simulink model "BMS_Full_Model"  (R2024a)
settings: Solver=VariableStepAuto  StartTime=0.0  StopTime=3600  RelTol=1e-3
undefined symbols (not defined in the file): Ion, Lithium
libraries: spsParallelRLCBranchLib x9, spsMosfetLib x9, spsBatteryLib x8, spsIdealSwitchLib x4, spsControlledCurrentSourceLib x1, spsDCVoltageSourceLib x1, spsDiodeLib x1, spsDCMachineLib x1, sps_lib x1, spsVoltageMeasurementLib x1
settings Model: Creator=kanna  LastModifiedBy=kanna

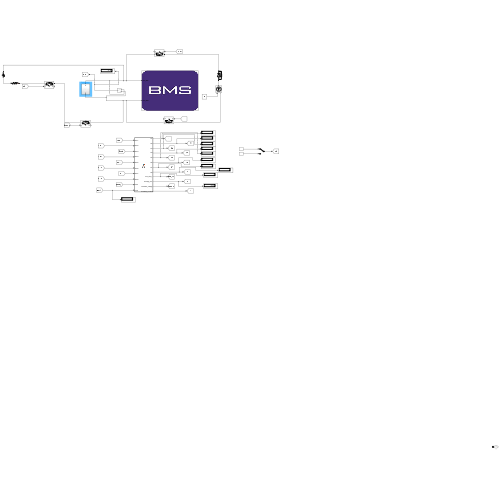
[thumbnail: Simulink's stored preview of the top-level diagram]
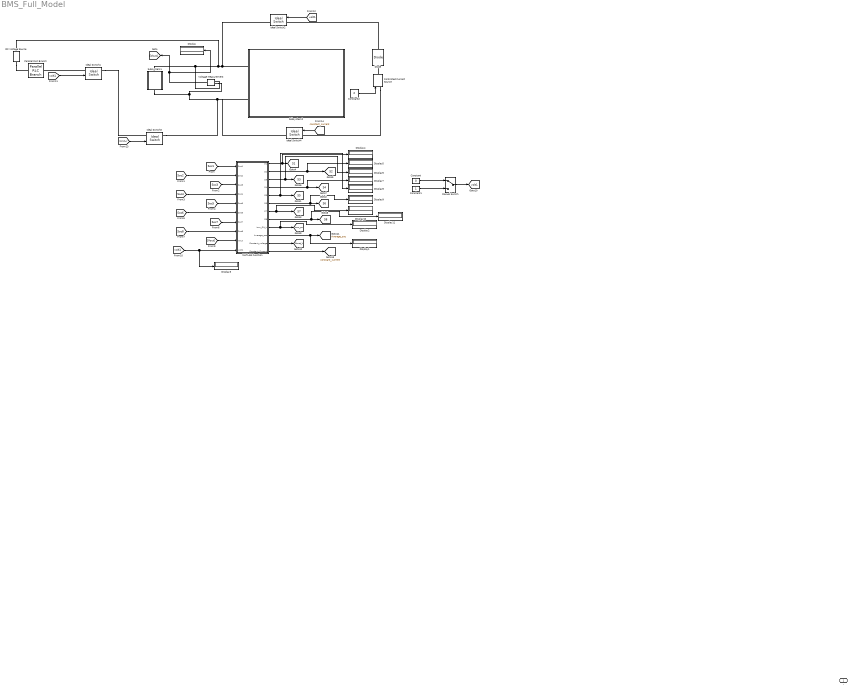
== system BMS_Full_Model ==
  Constant : Constant  Value=0
  Constant1 : Constant
  Constant2 : Constant  Value=2
  Controlled Current Source : spsControlledCurrentSourceLib/Controlled Current Source  Initialize=on  Source_Type=AC  Amplitude=0  Phase=0  Frequency=0  Measurements=None
  DC Voltage Source : spsDCVoltageSourceLib/DC Voltage Source  Amplitude=35  Measurements=None
  Diode : spsDiodeLib/Diode  Ron=0.001  Lon=0  Vf=0.8  IC=0  UseSnubber=0  Rs=500  Cs=250e-9  Measurements=off
  Display{,1..11} (12 alike) : Display
  Ideal Switch{1..4} (4 alike) : spsIdealSwitchLib/Ideal Switch  Ron=0.001  Lon=0  IC=0  Rs=1e5  Cs=inf  Measurements=on
  MATLAB Function : MATLAB Function  TreatAsAtomicUnit=on
  Manual Switch : ManualSwitch
  Parallel RLC Branch : spsParallelRLCBranchLib/Parallel RLC Branch  LConnTagsString=a  RConnTagsString=__new0  BranchType=R  Resistance=0.01  Inductance=1e-3  SetiL0=off  InitialCurrent=0  Capacitance=1e-6  Setx0=off  InitialVoltage=0  Measurements=None
  Subsystem1 : Subsystem
      settings: PortSchema="{\"entries\":[{\"content\":{\"sides\":[{\"content\":{},\"type\":\"ConnectorPlacement.EquallySpacedRectSide\",\"uuid\":\"ddaecf03-398d-4abe-ba2f-3d259c6a364a\"},{\"content\":{\"side\":\"RIGHT\"},\"type\":\"ConnectorPlacement.EquallySpacedRectSide\",\"uuid\":\"4de1636c-7844-41eb-a09b-b1e66b59fa18\"},{\"content\":{\"connectorIds\":[\"LConn1\"],\"side\":\"TOP\"},\"type\":\"ConnectorPlacement.EquallySpacedRectSide\",\"uuid\":\"76f54170-5ad1-4ec7-8870-ed8c99fdcc66\"},{\"content\":{\"connectorIds\":[\"RConn1\"],\"side\":\"BOTTOM\"},\"type\":\"ConnectorPlacement.EquallySpacedRectSide\",\"uuid\":\"75862763-7556-4715-9241-6073651da05c\"}]},\"type\":\"ConnectorPlacement.EquallySpacedConnector\",\"uuid\":\"7b1f8564-d695-4f68-8303-aa99595362ac\"}],\"packageUris\":[\"http://schema.mathworks.com/mf0/Connector/R2020b\"],\"version\":\"1.0\"}"
  Subsystem2 : Subsystem
      mask Display: image('GV4MPz3W8AAKAQj.jpeg');
  Voltage Measurement : spsVoltageMeasurementLib/Voltage Measurement  PhasorSimulation=off  OutputType=Complex  PSBequivalent=0
  - : PMIOPort  Side=Left
  tag scope: Average_soc=global, Const_V=global, S1=global, S2=global, S3=global, S4=global, S5=global, S6=global, S7=global, S8=global, constant_current=global, turn_on=global, volt1=global
  wires:
  MATLAB Function/1(S1) -> Display4/1, [S1]
  [Soc1] -> MATLAB Function/1(Soc1)
  [Soc2] -> MATLAB Function/2(Soc2)
  [Soc3] -> MATLAB Function/3(Soc3)
  [Soc4] -> MATLAB Function/4(Soc4)
  [Soc5] -> MATLAB Function/5(Soc5)
  [Soc6] -> MATLAB Function/6(Soc6)
  [Soc7] -> MATLAB Function/7(Soc7)
  [Soc8] -> MATLAB Function/8(Soc8)
  MATLAB Function/2(S2) -> Display5/1, [S2]
  MATLAB Function/3(S3) -> Display6/1, [S3]
  MATLAB Function/4(S4) -> Display7/1, [S4]
  MATLAB Function/5(S5) -> Display8/1, [S5]
  MATLAB Function/6(S6) -> Display9/1, [S6]
  MATLAB Function/7(S7) -> Display10/1, [S7]
  MATLAB Function/8(S8) -> Display11/1, [S8]
  Voltage Measurement/1 -> [Vout], Display/1
  [Vout] -> MATLAB Function/9(Vout)
  MATLAB Function/9(turn_ON_L) -> Display2/1, [turn_on]
  Constant/1 -> Manual Switch/1
  Constant1/1 -> Manual Switch/2
  [volt1] -> Ideal Switch1/1
  [volt1] -> Ideal Switch2/1
  MATLAB Function/10(Average_soc) -> Display1/1, [Average_soc]
  MATLAB Function/11(Constant_voltage) -> [Const_V]
  MATLAB Function/12(Constant_Current) -> [constant_current]
  [volt1] -> Display3/1, MATLAB Function/10(volt1)
  [Const_V] -> Ideal Switch3/1
  [constant_current] -> Ideal Switch4/1
  Manual Switch/1 -> [volt1]
  Constant2/1 -> Controlled Current Source/1
  connections:
  Ideal Switch1/LConn1 -- Parallel RLC Branch/LConn1
  DC Voltage Source/RConn1 -- Parallel RLC Branch/RConn1
  Ideal Switch2/RConn1 -- Subsystem2/LConn1 -- DC Voltage Source/LConn1 -- Subsystem1/RConn1 -- Voltage Measurement/LConn2
  Ideal Switch1/RConn1 -- Ideal Switch3/LConn1
  Controlled Current Source/LConn1 -- Ideal Switch4/LConn1
  Controlled Current Source/RConn1 -- Diode/LConn1
  Diode/RConn1 -- Ideal Switch2/LConn1
  Voltage Measurement/LConn1 -- Subsystem1/LConn1 -- Subsystem2/LConn2 -- Ideal Switch4/RConn1 -- Ideal Switch3/RConn1

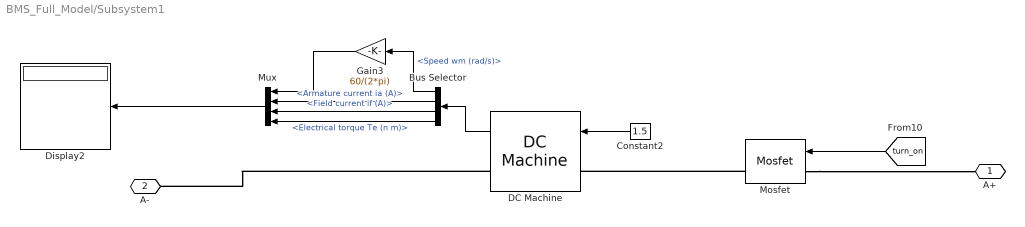
== system BMS_Full_Model/Subsystem1 ==
  Bus Selector : BusSelector  OutputSignals=Speed wm (rad/s),Armature current ia (A),Field current if (A),Electrical torque Te (n m)
  Constant2 : Constant  Value=1.5
  DC Machine : spsDCMachineLib/DC Machine  PresetModel=No  MechanicalLoad=Torque TL  FieldType=Permanent magnet  ShowDetailedParameters=on  MeasurementBus=off  RLa="[ 0.6  0.012]"  RLf="[ 240  120]"  Laf=1.8  MachineConstant=Torque constant (N.m/A)  Ke=1.8  Kt=1.8  J=1  Bm=0  Tf=0  w0=1  Ifinit=1.23834839145192e-21  TsPowergui=0  TsBlock=-1
  Display2 : Display
  Gain3 : Gain  Gain=60/(2*pi)
  Mosfet : spsMosfetLib/Mosfet  Ron=0.1  Lon=0  Rd=0.01  Vfd=0  IC=0  Rs=1e5  Cs=inf  Measurements=on
  Mux : Mux
  A+ : PMIOPort  Side=Left
  A- : PMIOPort  Port=2  Side=Right
  wires:
  Mux/1 -> Display2/1
  Gain3/1 -> Mux/1
  Bus Selector/4 -> Mux/4  "<Electrical torque Te (n m)>"
  Bus Selector/3 -> Mux/3  "<Field current if (A)>"
  Bus Selector/2 -> Mux/2  "<Armature current ia (A)>"
  Bus Selector/1 -> Gain3/1  "<Speed wm (rad/s)>"
  DC Machine/1 -> Bus Selector/1
  Constant2/1 -> DC Machine/1
  [turn_on] -> Mosfet/1
  connections:
  DC Machine/RConn1 -- A-/RConn1
  Mosfet/LConn1 -- A+/RConn1
  Mosfet/RConn1 -- DC Machine/LConn1

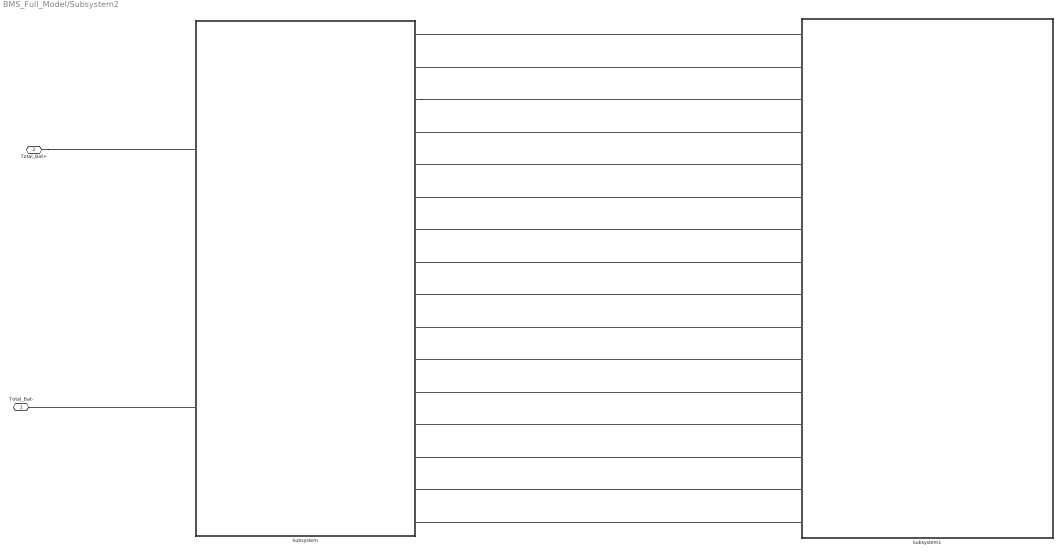
== system BMS_Full_Model/Subsystem2 ==
  Subsystem : Subsystem
  Subsystem1 : Subsystem
  Total_Bat- : PMIOPort  Side=Left
  Total_Bat+ : PMIOPort  Port=2  Side=Left
  connections:
  Total_Bat+/RConn1 -- Subsystem/LConn1
  Subsystem/LConn2 -- Total_Bat-/RConn1
  Subsystem1/LConn16 -- Subsystem/RConn16
  Subsystem1/LConn15 -- Subsystem/RConn15
  Subsystem1/LConn14 -- Subsystem/RConn14
  Subsystem1/LConn13 -- Subsystem/RConn13
  Subsystem1/LConn12 -- Subsystem/RConn12
  Subsystem1/LConn11 -- Subsystem/RConn11
  Subsystem1/LConn10 -- Subsystem/RConn10
  Subsystem1/LConn9 -- Subsystem/RConn9
  Subsystem1/LConn8 -- Subsystem/RConn8
  Subsystem1/LConn7 -- Subsystem/RConn7
  Subsystem1/LConn6 -- Subsystem/RConn6
  Subsystem1/LConn5 -- Subsystem/RConn5
  Subsystem1/LConn4 -- Subsystem/RConn4
  Subsystem1/LConn2 -- Subsystem/RConn2
  Subsystem1/LConn1 -- Subsystem/RConn1
  Subsystem/RConn3 -- Subsystem1/LConn3

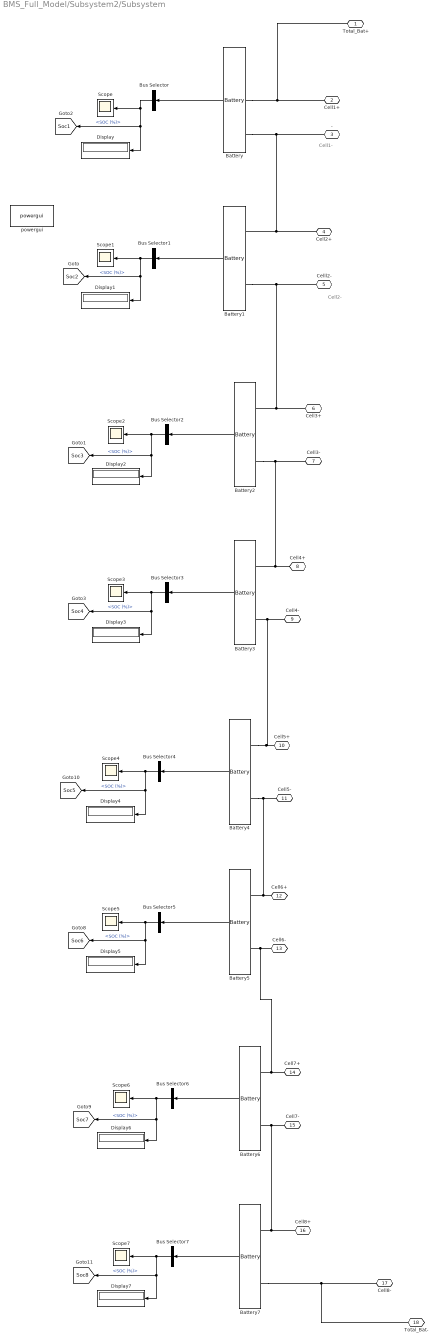
== system BMS_Full_Model/Subsystem2/Subsystem ==
  note: Cell2-
  note: Cell1-
  Battery : spsBatteryLib/Battery  BatType=Lithium-Ion  ShowTempParam=on  ThermalPreset="3.3V  2.3Ah  (LiFePO4)"  ShowAgeParam=off  NomV=3.3  NomQ=2.3  SOC=100  Batt_Tr=30  PresetModel=off  MaxQ=2.3  MinV=2.475  FullV=3.748  Dis_rate=2.3  R=0.014  Normal_OP=2.25  expZone="[3.4788       0.113]"  current=[6.5 13 32.5]  Units=Time  Tci=20  NomT=25  T2=0  MaxQ2=2.208  FullV2=3.45  Normal_OP2=2.85  expZone2="[3.22       0.015]"  Rca=0.6  ti=1000  Dp=0  Neq0=0  Tsim=1e6  Ta1=25  Qeol=5.4*0.9  Reol=0.013333*1.2  Char_age=[2.3478, 3]  Dis_age=[2.3478, 10]  N1=1500  N2=10500  N3=1000  N4=1400  Ta2=45  N5=950
  Battery{1..2,5..7} (5 alike) : spsBatteryLib/Battery  BatType=Lithium-Ion  ShowTempParam=off  ThermalPreset=no  ShowAgeParam=off  NomV=3.2  NomQ=18  SOC=100  Batt_Tr=30  PresetModel=on  MaxQ=18  MinV=2.4  FullV=3.7248  Dis_rate=7.8261  R=0.0017778  Normal_OP=16.2783  expZone="[3.4572     0.88435]"  current=[6.5 13 32.5]  Units=Time  Tci=20  NomT=20  T2=-30  MaxQ2=4.8  FullV2=7.1  Normal_OP2=5.655  expZone2="[6.58           1]"  Rca=0.6  ti=2000  Dp=0  Neq0=0  Tsim=1e6  Ta1=25  Qeol=5.4*0.9  Reol=0.013333*1.2  Char_age=[2.3478, 3]  Dis_age=[2.3478, 10]  N1=1500  N2=10500  N3=1000  N4=1400  Ta2=45  N5=950
  Battery3 : spsBatteryLib/Battery  BatType=Lithium-Ion  ShowTempParam=off  ThermalPreset=no  ShowAgeParam=off  NomV=3.2  NomQ=18  SOC=80  Batt_Tr=30  PresetModel=on  MaxQ=18  MinV=2.4  FullV=3.7248  Dis_rate=7.8261  R=0.0017778  Normal_OP=16.2783  expZone="[3.4572     0.88435]"  current=[6.5 13 32.5]  Units=Time  Tci=20  NomT=20  T2=-30  MaxQ2=4.8  FullV2=7.1  Normal_OP2=5.655  expZone2="[6.58           1]"  Rca=0.6  ti=2000  Dp=0  Neq0=0  Tsim=1e6  Ta1=25  Qeol=5.4*0.9  Reol=0.013333*1.2  Char_age=[2.3478, 3]  Dis_age=[2.3478, 10]  N1=1500  N2=10500  N3=1000  N4=1400  Ta2=45  N5=950
  Battery4 : spsBatteryLib/Battery  BatType=Lithium-Ion  ShowTempParam=off  ThermalPreset=no  ShowAgeParam=off  NomV=3.2  NomQ=18  SOC=90  Batt_Tr=30  PresetModel=on  MaxQ=18  MinV=2.4  FullV=3.7248  Dis_rate=7.8261  R=0.0017778  Normal_OP=16.2783  expZone="[3.4572     0.88435]"  current=[6.5 13 32.5]  Units=Time  Tci=20  NomT=20  T2=-30  MaxQ2=4.8  FullV2=7.1  Normal_OP2=5.655  expZone2="[6.58           1]"  Rca=0.6  ti=2000  Dp=0  Neq0=0  Tsim=1e6  Ta1=25  Qeol=5.4*0.9  Reol=0.013333*1.2  Char_age=[2.3478, 3]  Dis_age=[2.3478, 10]  N1=1500  N2=10500  N3=1000  N4=1400  Ta2=45  N5=950
  Bus Selector{,1..7} (8 alike) : BusSelector  OutputSignals=SOC (%)
  Display{,1..7} (8 alike) : Display
  Scope{,1..7} (8 alike) : Scope
  powergui : sps_lib/powergui  Priority=1  SimulationMode=Discrete  SampleTime=10000e-6  frequency=60  Iterations=50  frequencyindice=0  Pbase=100e6  ErrMax=1e-4  UnitsV=kV  UnitsW=MW  buscounter=0  FunctionMessages=off  echomessages=off  EnableUseOfTLC=off  CurrentSourceSwitches=off  DisableSnubberDevices=off  DisableRonSwitches=off  DisableVfSwitches=off  DisplayEquations=off  AutomaticDiscreteSolvers=off  SolverType=Tustin/Backward Euler (TBE)  Interpol=off  ExternalGateDelay=off  methode=off  Ts=100  x0status=blocks  SPID=on  SwTol=0  HookPort=off  NonlinearTolerance=1e-4  nMaxIteration=100  ContinueOnMaxIteration=off  RestoreLinks=warning  ResistiveCurrentMeasurement=off  Frange=[0:2:500]  Ylog=off  Xlog=on  ShowGrid=off  save=off  variable=ZData  structure=0  ZoomFFT=off  StartTime=0.0  cycles=1  DisplayStyle=1  fundamental=60  FreqAxis=off  MaxFrequency=1000  frequencyindicesteady=1  RmsSteady=1  display=off
  Total_Bat+ : PMIOPort  Side=Left
  Cell1+ : PMIOPort  Port=2  Side=Right
  - : PMIOPort  Port=3  Side=Right
  Cell2+ : PMIOPort  Port=4  Side=Right
  Celll2- : PMIOPort  Port=5  Side=Right
  Cell3+ : PMIOPort  Port=6  Side=Right
  Cell3- : PMIOPort  Port=7  Side=Right
  Cell4+ : PMIOPort  Port=8  Side=Right
  Cell4- : PMIOPort  Port=9  Side=Right
  Cell5+ : PMIOPort  Port=10  Side=Right
  Cell5- : PMIOPort  Port=11  Side=Right
  Cell6+ : PMIOPort  Port=12  Side=Right
  Cell6- : PMIOPort  Port=13  Side=Right
  Cell7+ : PMIOPort  Port=14  Side=Right
  Cell7- : PMIOPort  Port=15  Side=Right
  Cell8+ : PMIOPort  Port=16  Side=Right
  Cell8- : PMIOPort  Port=17  Side=Right
  Total_Bat- : PMIOPort  Port=18  Side=Left
  tag scope: Soc1=global, Soc2=global, Soc3=global, Soc4=global, Soc5=global, Soc6=global, Soc7=global, Soc8=global
  wires:
  Battery4/1 -> Bus Selector4/1
  Bus Selector6/1 -> [Soc7], Display6/1, Scope6/1  "<SOC (%)>"
  Bus Selector2/1 -> [Soc3], Display2/1, Scope2/1  "<SOC (%)>"
  Bus Selector7/1 -> Scope7/1, Display7/1, [Soc8]  "<SOC (%)>"
  Bus Selector4/1 -> [Soc5], Display4/1, Scope4/1  "<SOC (%)>"
  Bus Selector5/1 -> Scope5/1, Display5/1, [Soc6]  "<SOC (%)>"
  Bus Selector1/1 -> Scope1/1, Display1/1, [Soc2]  "<SOC (%)>"
  Bus Selector3/1 -> Scope3/1, Display3/1, [Soc4]  "<SOC (%)>"
  Bus Selector/1 -> [Soc1], Display/1, Scope/1  "<SOC (%)>"
  Battery3/1 -> Bus Selector3/1
  Battery7/1 -> Bus Selector7/1
  Battery/1 -> Bus Selector/1
  Battery1/1 -> Bus Selector1/1
  Battery2/1 -> Bus Selector2/1
  Battery6/1 -> Bus Selector6/1
  Battery5/1 -> Bus Selector5/1
  connections:
  Cell6-/RConn1 -- Battery5/LConn2 -- Battery6/LConn1 -- Cell7+/RConn1
  Battery/LConn1 -- Total_Bat+/RConn1 -- Cell1+/RConn1
  Battery7/LConn2 -- Total_Bat-/RConn1 -- Cell8-/RConn1
  Cell7-/RConn1 -- Battery7/LConn1 -- Cell8+/RConn1 -- Battery6/LConn2
  Battery2/LConn2 -- Battery3/LConn1 -- Cell4+/RConn1 -- Cell3-/RConn1
  Cell4-/RConn1 -- Battery4/LConn1 -- Cell5+/RConn1 -- Battery3/LConn2
  Battery/LConn2 -- Battery1/LConn1 -- Cell2+/RConn1 -- -/RConn1
  Battery1/LConn2 -- Battery2/LConn1 -- Cell3+/RConn1 -- Celll2-/RConn1
  Battery4/LConn2 -- Battery5/LConn1 -- Cell6+/RConn1 -- Cell5-/RConn1

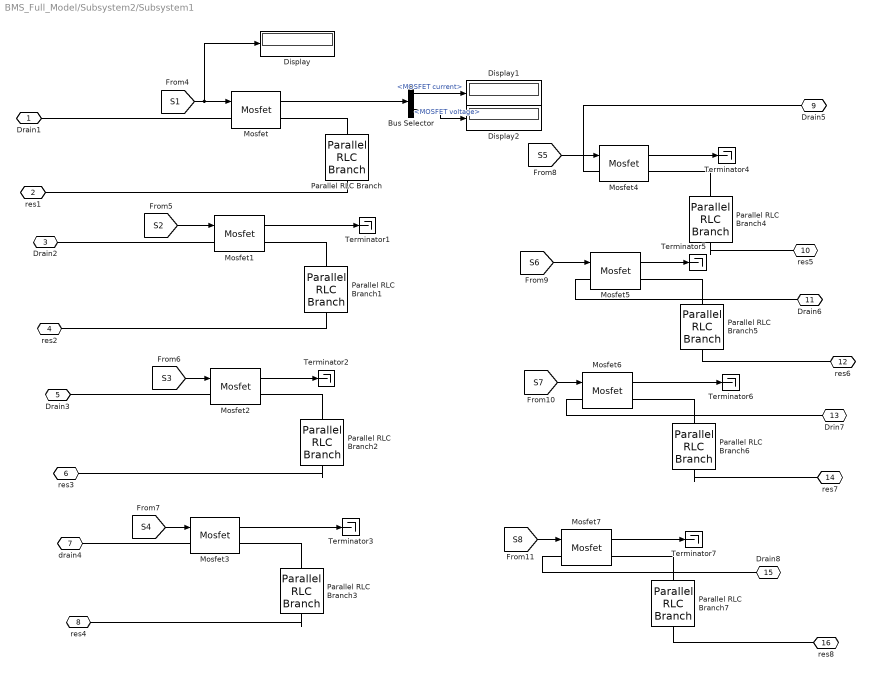
== system BMS_Full_Model/Subsystem2/Subsystem1 ==
  Bus Selector : BusSelector  OutputSignals=MOSFET current,MOSFET voltage
  Display : Display
  Display1 : Display
  Display2 : Display
  Mosfet{,1..7} (8 alike) : spsMosfetLib/Mosfet  Ron=0.1  Lon=0  Rd=0.01  Vfd=0  IC=0  Rs=1e5  Cs=inf  Measurements=on
  Parallel RLC Branch{,1..7} (8 alike) : spsParallelRLCBranchLib/Parallel RLC Branch  LConnTagsString=a  RConnTagsString=__new0  BranchType=R  Resistance=1  Inductance=1e-3  SetiL0=off  InitialCurrent=0  Capacitance=1e-6  Setx0=off  InitialVoltage=0  Measurements=None
  Terminator{1..7} (7 alike) : Terminator
  Drain1 : PMIOPort  Side=Left
  res1 : PMIOPort  Port=2  Side=Left
  Drain2 : PMIOPort  Port=3  Side=Left
  res2 : PMIOPort  Port=4  Side=Left
  Drain3 : PMIOPort  Port=5  Side=Left
  res3 : PMIOPort  Port=6  Side=Left
  drain4 : PMIOPort  Port=7  Side=Left
  res4 : PMIOPort  Port=8  Side=Left
  Drain5 : PMIOPort  Port=9  Side=Left
  res5 : PMIOPort  Port=10  Side=Left
  Drain6 : PMIOPort  Port=11  Side=Left
  res6 : PMIOPort  Port=12  Side=Left
  Drin7 : PMIOPort  Port=13  Side=Left
  res7 : PMIOPort  Port=14  Side=Left
  Drain8 : PMIOPort  Port=15  Side=Left
  res8 : PMIOPort  Port=16  Side=Left
  wires:
  [S1] -> Display/1, Mosfet/1
  [S3] -> Mosfet2/1
  [S5] -> Mosfet4/1
  Mosfet2/1 -> Terminator2/1
  Mosfet6/1 -> Terminator6/1
  Mosfet3/1 -> Terminator3/1
  [S2] -> Mosfet1/1
  [S4] -> Mosfet3/1
  [S6] -> Mosfet5/1
  [S7] -> Mosfet6/1
  [S8] -> Mosfet7/1
  Mosfet1/1 -> Terminator1/1
  Mosfet/1 -> Bus Selector/1
  Mosfet4/1 -> Terminator4/1
  Mosfet5/1 -> Terminator5/1
  Mosfet7/1 -> Terminator7/1
  Bus Selector/1 -> Display1/1  "<MOSFET current>"
  Bus Selector/2 -> Display2/1  "<MOSFET voltage>"
  connections:
  Mosfet2/LConn1 -- Drain3/RConn1
  Parallel RLC Branch2/RConn1 -- res3/RConn1
  Mosfet3/RConn1 -- Parallel RLC Branch3/LConn1
  Mosfet1/RConn1 -- Parallel RLC Branch1/LConn1
  Mosfet5/RConn1 -- Parallel RLC Branch5/LConn1
  Mosfet2/RConn1 -- Parallel RLC Branch2/LConn1
  Parallel RLC Branch3/RConn1 -- res4/RConn1
  Mosfet7/RConn1 -- Parallel RLC Branch7/LConn1
  Mosfet6/RConn1 -- Parallel RLC Branch6/LConn1
  Mosfet4/RConn1 -- Parallel RLC Branch4/LConn1
  Parallel RLC Branch6/RConn1 -- res7/RConn1
  Mosfet7/LConn1 -- Drain8/RConn1
  Mosfet1/LConn1 -- Drain2/RConn1
  Parallel RLC Branch/RConn1 -- res1/RConn1
  Parallel RLC Branch4/RConn1 -- res5/RConn1
  Mosfet3/LConn1 -- drain4/RConn1
  Parallel RLC Branch1/RConn1 -- res2/RConn1
  Parallel RLC Branch5/RConn1 -- res6/RConn1
  Parallel RLC Branch7/RConn1 -- res8/RConn1
  Mosfet5/LConn1 -- Drain6/RConn1
  Mosfet6/LConn1 -- Drin7/RConn1
  Mosfet4/LConn1 -- Drain5/RConn1
  Parallel RLC Branch/LConn1 -- Mosfet/RConn1
  Drain1/RConn1 -- Mosfet/LConn1

== matlab function BMS_Full_Model/MATLAB Function ==
  data: S1 output; Soc1 input; Soc2 input; Soc3 input; Soc4 input; Soc5 input; Soc6 input; Soc7 input; Soc8 input; Vout input; volt1 input; S2 output; S3 output; S4 output; S5 output; S6 output; S7 output; S8 output; turn_ON_L output; Average_soc output; Constant_voltage output; Constant_Current output
function [S1, S2, S3, S4, S5, S6, S7, S8, turn_ON_L, Average_soc, Constant_voltage, Constant_Current] = BMS(Soc1, Soc2, Soc3, Soc4, Soc5, Soc6, Soc7, Soc8, Vout, volt1)
    [Constant_voltage, Constant_Current,turn_ON_L ] = deal(0); % Default value
    [S1, S2, S3, S4, S5, S6, S7, S8] = deal(1);
    

    % Average Soc function
    Average_soc = Avg_soc(Soc1, Soc2, Soc3, Soc4, Soc5, Soc6, Soc7, Soc8);

   % if all(soc~= min(soc))
    % Call Cell_balencing function
    % Convert to integers

    sw =[S1, S2, S3, S4, S5, S6, S7, S8];

    if all(sw~=0)
    SocArray = int32([Soc1, Soc2, Soc3, Soc4, Soc5, Soc6, Soc7, Soc8]);


    % Initialize Switch array
    Switch_sel = zeros(1,8);

    % Find the minimum SoC
    min_soc = min(SocArray);
      max_soc=max(SocArray); 
      disp('max_soc:');
    disp(max_soc);
    

    % Perform cell balancing
   
    for i = 1:length(SocArray)
        if SocArray(i) > min_soc
            Switch_sel(i) = 1;
        elseif SocArray(i) <= min_soc
            Switch_sel(i) = 0;
        end
 

    % Assign outputs
 S1= Switch_sel(1);
 S2= Switch_sel(2);
 S3= Switch_sel(3);
 S4= Switch_sel(4);
 S5= Switch_sel(5);
 S6= Switch_sel(6);
 S7= Switch_sel(7);
 S8= Switch_sel(8);

    end

    %end

    else 

    % Call operatingvolt function
    V_operating = operatingvolt(Vout);

    % Call Chargingvolt function
    charging = Chargingvolt(volt1);

    % To turn ON current or Voltage source
    if Average_soc > 80 && Average_soc <= 100
        Constant_voltage = 1;
        Constant_Current = 0;
    elseif Average_soc <= 80
        Constant_Current = 1;
        Constant_voltage = 0;
    end

    % To turn ON or OFF load
    if V_operating && charging
        turn_ON_L = 1;
    else
        turn_ON_L = 0;
    end

    % Display the results
    disp('turn_ON_L:');
    disp(turn_ON_L);
    disp('Average_soc:');
    disp(Average_soc);
    disp('Constant_voltage:');
    disp(Constant_voltage);
    disp('Constant_Current:');
    disp(Constant_Current);
    end
   

   

function V_operating = operatingvolt(Vout)
    V_max = 30;
    V_min = 22;
    Vout = int16(Vout);
    if Vout < V_max && Vout > V_min
        V_operating = 1;
    else
        V_operating = 0;
    end
end

function charging = Chargingvolt(volt1)
    if volt1 == 1
        charging = 0;
    else
        charging = 1;
    end
end

function Average_soc = Avg_soc(Soc1, Soc2, Soc3, Soc4, Soc5, Soc6, Soc7, Soc8)
    Avg_soc = [Soc1, Soc2, Soc3, Soc4, Soc5, Soc6, Soc7, Soc8];
    Average_soc = mean(Avg_soc);
end
end
